simulink model "Top_Model"  (R2020b)
settings: Solver=FixedStepAuto  StartTime=0.0  StopTime=TMax  FixedStep=DT  RelTol=1e-3
undefined symbols (not defined in the file): OutList, strmatch
settings Model: Creator=lpwoolcock  LastModifiedBy=lpwoolcock

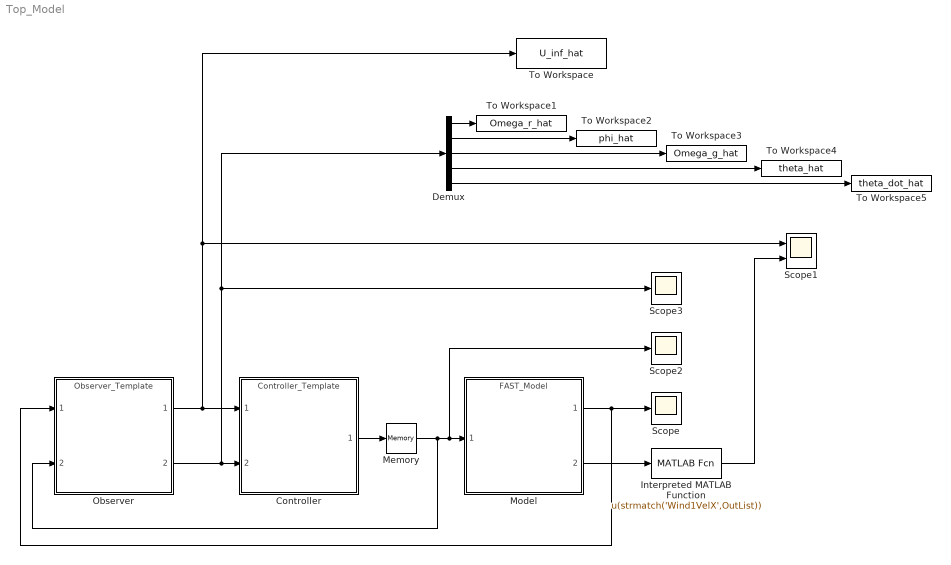
== system Top_Model ==
  Controller : ModelReference  ModelNameDialog=Controller_Template.slx  SimulationMode=Normal  ModelReferenceVersion=1.36
  Demux : Demux  Outputs=5
  Interpreted MATLAB Function : MATLABFcn  MATLABFcn=u(strmatch('Wind1VelX',OutList))
  Memory : Memory  InitialCondition=zeros(2,1)
  Model : ModelReference  ModelNameDialog=FAST_Model.slx  SimulationMode=Normal  ModelReferenceVersion=1.21
  Observer : ModelReference  ModelNameDialog=Observer_Template.slx  SimulationMode=Normal  ModelReferenceVersion=1.31
  Scope : Scope
  Scope1 : Scope  NumInputPorts=2
  Scope2 : Scope
  Scope3 : Scope
  To Workspace : ToWorkspace  VariableName=U_inf_hat  SaveFormat=Timeseries  SampleTime=-1
  To Workspace1 : ToWorkspace  VariableName=Omega_r_hat  SaveFormat=Timeseries  SampleTime=-1
  To Workspace2 : ToWorkspace  VariableName=phi_hat  SaveFormat=Timeseries  SampleTime=-1
  To Workspace3 : ToWorkspace  VariableName=Omega_g_hat  SaveFormat=Timeseries  SampleTime=-1
  To Workspace4 : ToWorkspace  VariableName=theta_hat  SaveFormat=Timeseries  SampleTime=-1
  To Workspace5 : ToWorkspace  VariableName=theta_dot_hat  SaveFormat=Timeseries  SampleTime=-1
  wires:
  Model/1 -> Observer/1, Scope/1
  Model/2 -> Interpreted MATLAB Function/1
  Interpreted MATLAB Function/1 -> Scope1/2
  Controller/1 -> Memory/1
  Observer/1 -> Controller/1, Scope1/1, To Workspace/1
  Observer/2 -> Controller/2, Scope3/1, Demux/1
  Demux/1 -> To Workspace1/1
  Demux/2 -> To Workspace2/1
  Demux/3 -> To Workspace3/1
  Demux/4 -> To Workspace4/1
  Demux/5 -> To Workspace5/1
  Memory/1 -> Model/1, Scope2/1, Observer/2
